simulink model "SISO_Sliding_Mode_Controlx_beta_first"  (R2021b)
settings: Solver=VariableStepAuto  StartTime=tspan(1)  StopTime=tspan(2)  RelTol=1e-8
undefined symbols (not defined in the file): BL_gain, K_switch, lambda_1_num, lambda_2_num, r_sim, Tau, y1_0, y2_0
libraries: simulink x2, simulink_extras x1
settings Model: Creator=domin  LastModifiedBy=domin
settings SolverCC: AlgebraicLoopSolver=TrustRegion
settings DebuggingCC: SFMachineParentedDataDiag=warning

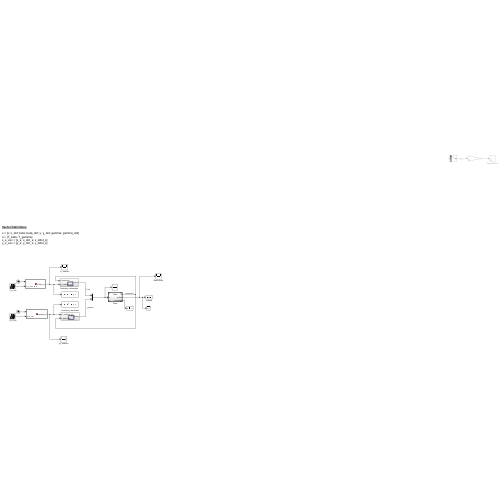
[thumbnail: Simulink's stored preview of the top-level diagram]
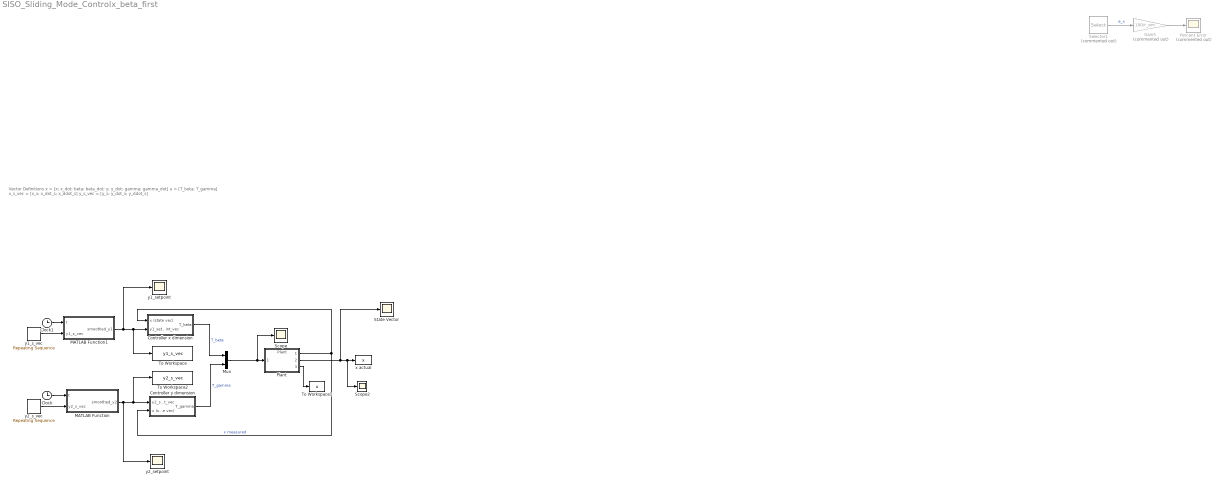
== system SISO_Sliding_Mode_Controlx_beta_first ==
  note: Vector Definitions
      |
      | x = [x; x_dot; beta; beta_dot; y; y_dot; gamma; gamma_dot]
      | u = [T_beta; T_gamma]
      | x_s_vec = [x_s; x_dot_s; x_ddot_s]
      | y_s_vec = [y_s; y_dot_s; y_ddot_s]
  Clock : Clock
  Clock1 : Clock
  Controller x dimension : Subsystem
  Controller y dimension : Subsystem
  Gain5 : Gain  Commented=on  Gain=100/r_sim
  MATLAB Function : MATLAB Function  TreatAsAtomicUnit=on
  MATLAB Function1 : MATLAB Function  TreatAsAtomicUnit=on
  Mux : Mux  Inputs=2
  Percent Error : Scope  Commented=on
  Plant : ModelReference  ModelNameDialog=Plant  SimulationMode=Normal  ModelReferenceVersion=1.107
  Scope : Scope
  Scope2 : Scope
  Selector1 : Selector  Commented=on  InputPortWidth=5  IndexOptions=Index vector (dialog)  Indices=[1]  OutputSizes=1
  State Vector : Scope
  To Workspace : ToWorkspace  VariableName=y1_s_vec  SampleTime=-1
  To Workspace1 : ToWorkspace  VariableName=u  SampleTime=-1
  To Workspace2 : ToWorkspace  VariableName=y2_s_vec  SampleTime=-1
  x actual : ToWorkspace  VariableName=x  SampleTime=-1
  y1_s_vec : simulink/Sources/Repeating Sequence  rep_seq_t=beta_BVP_sol.x'  rep_seq_y=y_s_vec_new
  y1_setpoint : Scope
  y2_s_vec : simulink/Sources/Repeating Sequence  rep_seq_t=beta_BVP_sol.x'  rep_seq_y=y_s_vec_new
  y2_setpoint : Scope
  wires:
  Gain5/1 -> Percent Error/1
  Selector1/1 -> Gain5/1  "e_x"
  Controller x dimension/1(T_beta) -> Mux/1  "T_beta"
  Controller y dimension/1(T_gamma) -> Mux/2  "T_gamma"
  Mux/1 -> Plant/1, Scope/1
  Plant/1 -> Controller x dimension/1(x (state vec)), Controller y dimension/2(x (state vec))  "x measured"
  Plant/2 -> State Vector/1, x actual/1, Scope2/1
  Plant/3 -> To Workspace1/1
  MATLAB Function/1(smoothed_y2) -> y2_setpoint/1, To Workspace2/1, Controller y dimension/1(y2_setpoint_vec)
  Clock/1 -> MATLAB Function/1(t)
  y2_s_vec/1 -> MATLAB Function/2(y2_s_vec)
  Clock1/1 -> MATLAB Function1/1(t)
  y1_s_vec/1 -> MATLAB Function1/2(y1_s_vec)
  MATLAB Function1/1(smoothed_y1) -> y1_setpoint/1, To Workspace/1, Controller x dimension/2(y1_setpoint_vec)

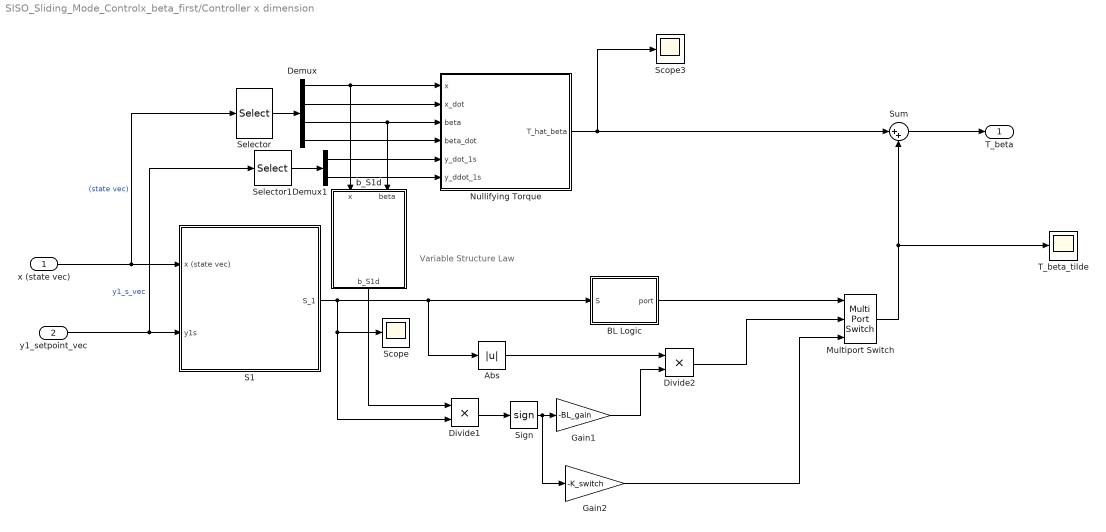
== system SISO_Sliding_Mode_Controlx_beta_first/Controller x dimension ==
  note: Variable Structure Law
  x (state vec) : Inport
  y1_setpoint_vec : Inport  Port=2
  Abs : Abs
  BL Logic : MATLAB Function  TreatAsAtomicUnit=on
  Demux : Demux
  Demux1 : Demux  Outputs=2
  Divide1 : Product  Inputs=**
  Divide2 : Product  Inputs=**
  Gain1 : Gain  Gain=-BL_gain
  Gain2 : Gain  Gain=-K_switch
  Multiport Switch : MultiPortSwitch  Inputs=2
  Nullifying Torque : MATLAB Function  TreatAsAtomicUnit=on
  S1 : Subsystem
  Scope : Scope
  Scope3 : Scope
  Selector : Selector  InputPortWidth=8  IndexOptions=Index vector (dialog)  Indices=[1:4]  OutputSizes=1
  Selector1 : Selector  InputPortWidth=3  IndexOptions=Index vector (dialog)  Indices=[2 3]  OutputSizes=1
  Sign : Signum
  Sum : Sum  Inputs=|++
  T_beta_tilde : Scope
  b_S1d : MATLAB Function  TreatAsAtomicUnit=on
  T_beta : Outport
  wires:
  Sum/1 -> T_beta/1
  x (state vec)/1 -> Selector/1, S1/1(x (state vec))  "(state vec)"
  y1_setpoint_vec/1 -> Selector1/1, S1/2(y1s)  "y1_s_vec"
  Selector/1 -> Demux/1
  Demux/2 -> Nullifying Torque/2(x_dot)
  Demux/4 -> Nullifying Torque/4(beta_dot)
  Selector1/1 -> Demux1/1
  Demux1/1 -> Nullifying Torque/5(y_dot_1s)
  Demux1/2 -> Nullifying Torque/6(y_ddot_1s)
  Nullifying Torque/1(T_hat_beta) -> Scope3/1, Sum/1
  b_S1d/1(b_S1d) -> Divide1/1
  Divide2/1 -> Multiport Switch/2
  S1/1(S_1) -> Divide1/2, Scope/1, Abs/1, BL Logic/1(S)
  Demux/3 -> Nullifying Torque/3(beta), b_S1d/2(beta)
  Demux/1 -> Nullifying Torque/1(x), b_S1d/1(x)
  Gain1/1 -> Divide2/2
  BL Logic/1(port) -> Multiport Switch/1
  Multiport Switch/1 -> Sum/2, T_beta_tilde/1
  Sign/1 -> Gain2/1, Gain1/1
  Divide1/1 -> Sign/1
  Gain2/1 -> Multiport Switch/3
  Abs/1 -> Divide2/1

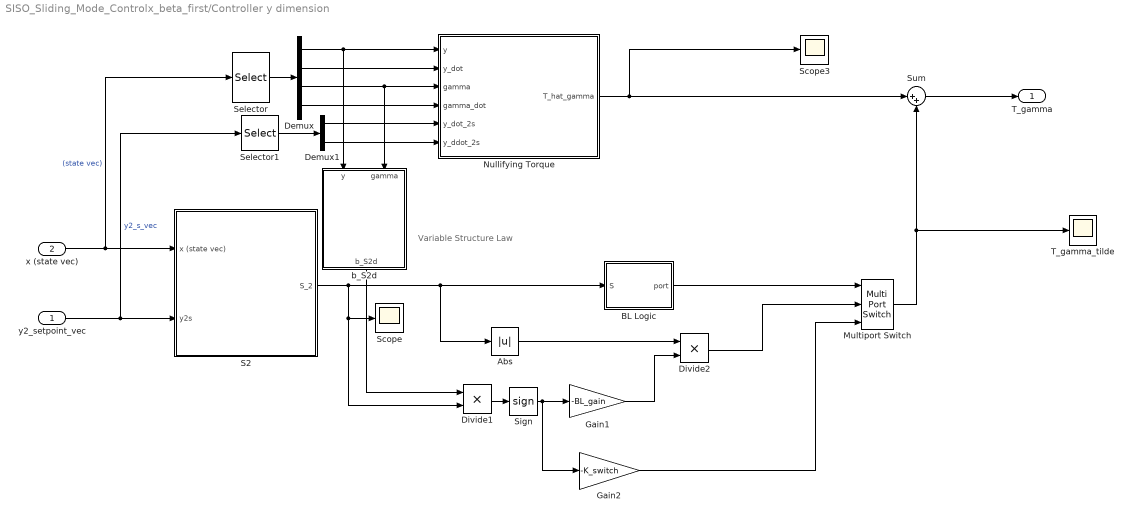
== system SISO_Sliding_Mode_Controlx_beta_first/Controller y dimension ==
  note: Variable Structure Law
  y2_setpoint_vec : Inport
  x (state vec) : Inport  Port=2
  Abs : Abs
  BL Logic : MATLAB Function  TreatAsAtomicUnit=on
  Demux : Demux
  Demux1 : Demux  Outputs=2
  Divide1 : Product  Inputs=**
  Divide2 : Product  Inputs=**
  Gain1 : Gain  Gain=-BL_gain
  Gain2 : Gain  Gain=-K_switch
  Multiport Switch : MultiPortSwitch  Inputs=2
  Nullifying Torque : MATLAB Function  TreatAsAtomicUnit=on
  S2 : Subsystem
  Scope : Scope
  Scope3 : Scope
  Selector : Selector  InputPortWidth=8  IndexOptions=Index vector (dialog)  Indices=[5:8]  OutputSizes=1
  Selector1 : Selector  InputPortWidth=3  IndexOptions=Index vector (dialog)  Indices=[2 3]  OutputSizes=1
  Sign : Signum
  Sum : Sum  Inputs=|++
  T_gamma_tilde : Scope
  b_S2d : MATLAB Function  TreatAsAtomicUnit=on
  T_gamma : Outport
  wires:
  Demux/2 -> Nullifying Torque/2(y_dot)
  Nullifying Torque/1(T_hat_gamma) -> Scope3/1, Sum/1
  Demux1/1 -> Nullifying Torque/5(y_dot_2s)
  Selector/1 -> Demux/1
  Demux/4 -> Nullifying Torque/4(gamma_dot)
  Selector1/1 -> Demux1/1
  Demux1/2 -> Nullifying Torque/6(y_ddot_2s)
  x (state vec)/1 -> Selector/1, S2/1(x (state vec))  "(state vec)"
  y2_setpoint_vec/1 -> S2/2(y2s), Selector1/1  "y2_s_vec"
  Sum/1 -> T_gamma/1
  Demux/3 -> Nullifying Torque/3(gamma), b_S2d/2(gamma)
  Demux/1 -> Nullifying Torque/1(y), b_S2d/1(y)
  Gain1/1 -> Divide2/2
  Abs/1 -> Divide2/1
  Gain2/1 -> Multiport Switch/3
  Multiport Switch/1 -> Sum/2, T_gamma_tilde/1
  BL Logic/1(port) -> Multiport Switch/1
  Sign/1 -> Gain1/1, Gain2/1
  b_S2d/1(b_S2d) -> Divide1/1
  Divide2/1 -> Multiport Switch/2
  S2/1(S_2) -> Abs/1, BL Logic/1(S), Divide1/2, Scope/1
  Divide1/1 -> Sign/1

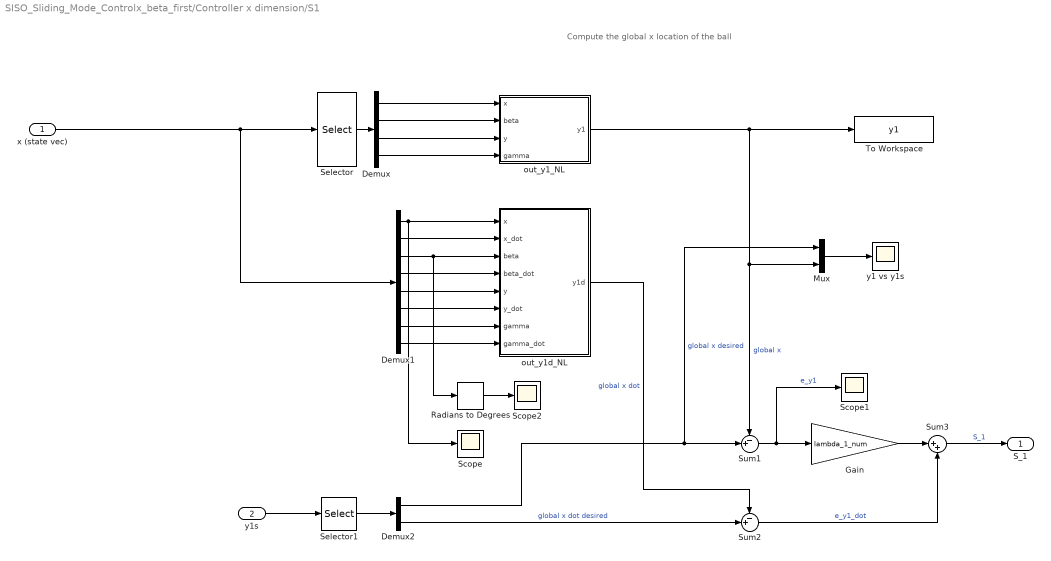
== system SISO_Sliding_Mode_Controlx_beta_first/Controller x dimension/S1 ==
  note: Compute the global x location of the ball
  x (state vec) : Inport
  y1s : Inport  Port=2
  Demux : Demux
  Demux1 : Demux  Outputs=8
  Demux2 : Demux  Outputs=2
  Gain : Gain  Gain=lambda_1_num
  Mux : Mux  Inputs=2
  Radians to Degrees : simulink_extras/Transformations/Radians to Degrees
  Scope : Scope
  Scope1 : Scope
  Scope2 : Scope
  Selector : Selector  InputPortWidth=8  IndexOptions=Index vector (dialog)  Indices=[1 3 5 7]  OutputSizes=1
  Selector1 : Selector  InputPortWidth=3  IndexOptions=Index vector (dialog)  Indices=[1 2]  OutputSizes=1
  Sum1 : Sum  Inputs=-+|
  Sum2 : Sum  Inputs=-+|
  Sum3 : Sum  Inputs=|++
  To Workspace : ToWorkspace  VariableName=y1  SampleTime=-1
  out_y1_NL : MATLAB Function  TreatAsAtomicUnit=on
  out_y1d_NL : MATLAB Function  TreatAsAtomicUnit=on
  y1 vs y1s : Scope
  S_1 : Outport
  wires:
  Demux/4 -> out_y1_NL/4(gamma)
  Sum3/1 -> S_1/1  "S_1"
  Selector/1 -> Demux/1
  Demux1/5 -> out_y1d_NL/5(y)
  Demux1/1 -> Scope/1, out_y1d_NL/1(x)
  Demux1/4 -> out_y1d_NL/4(beta_dot)
  Demux/2 -> out_y1_NL/2(beta)
  Sum1/1 -> Scope1/1, Gain/1  "e_y1"
  Sum2/1 -> Sum3/2  "e_y1_dot"
  x (state vec)/1 -> Demux1/1, Selector/1
  Gain/1 -> Sum3/1
  Demux/1 -> out_y1_NL/1(x)
  Demux/3 -> out_y1_NL/3(y)
  Demux1/2 -> out_y1d_NL/2(x_dot)
  Demux1/6 -> out_y1d_NL/6(y_dot)
  Demux1/8 -> out_y1d_NL/8(gamma_dot)
  out_y1_NL/1(y1) -> Mux/2, Sum1/1, To Workspace/1  "global x"
  Demux1/7 -> out_y1d_NL/7(gamma)
  Demux2/1 -> Mux/1, Sum1/2  "global x desired"
  Demux1/3 -> Radians to Degrees/1, out_y1d_NL/3(beta)
  Demux2/2 -> Sum2/2  "global x dot desired"
  y1s/1 -> Selector1/1
  out_y1d_NL/1(y1d) -> Sum2/1  "global x dot"
  Selector1/1 -> Demux2/1
  Mux/1 -> y1 vs y1s/1
  Radians to Degrees/1 -> Scope2/1

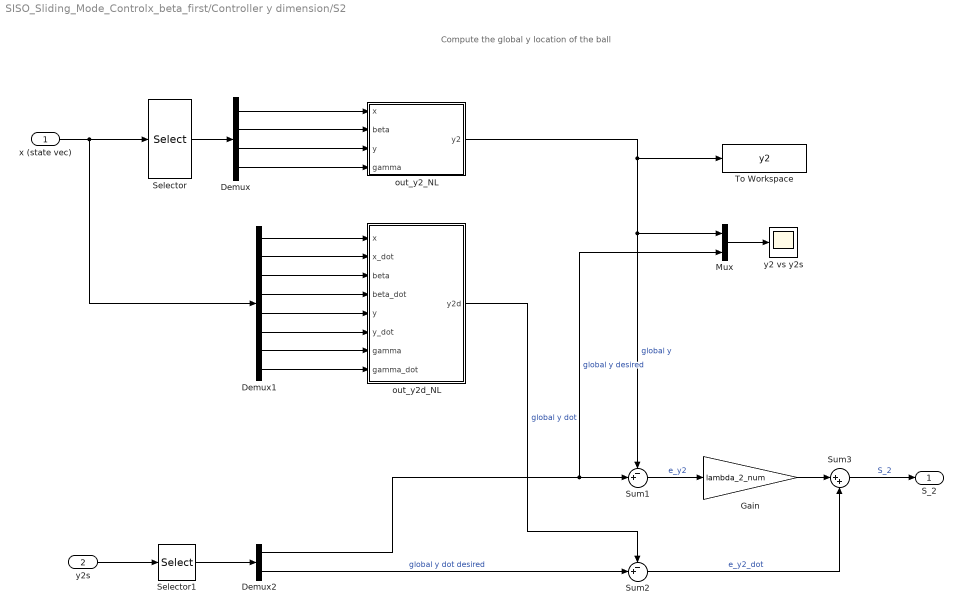
== system SISO_Sliding_Mode_Controlx_beta_first/Controller y dimension/S2 ==
  note: Compute the global y location of the ball
  x (state vec) : Inport
  y2s : Inport  Port=2
  Demux : Demux
  Demux1 : Demux  Outputs=8
  Demux2 : Demux  Outputs=2
  Gain : Gain  Gain=lambda_2_num
  Mux : Mux  Inputs=2
  Selector : Selector  InputPortWidth=8  IndexOptions=Index vector (dialog)  Indices=[1 3 5 7]  OutputSizes=1
  Selector1 : Selector  InputPortWidth=3  IndexOptions=Index vector (dialog)  Indices=[1 2]  OutputSizes=1
  Sum1 : Sum  Inputs=-+|
  Sum2 : Sum  Inputs=-+|
  Sum3 : Sum  Inputs=|++
  To Workspace : ToWorkspace  VariableName=y2  SampleTime=-1
  out_y2_NL : MATLAB Function  TreatAsAtomicUnit=on
  out_y2d_NL : MATLAB Function  TreatAsAtomicUnit=on
  y2 vs y2s : Scope
  S_2 : Outport
  wires:
  Demux/4 -> out_y2_NL/4(gamma)
  Sum3/1 -> S_2/1  "S_2"
  Selector/1 -> Demux/1
  Demux1/5 -> out_y2d_NL/5(y)
  Demux1/1 -> out_y2d_NL/1(x)
  Demux1/4 -> out_y2d_NL/4(beta_dot)
  Demux/2 -> out_y2_NL/2(beta)
  Sum1/1 -> Gain/1  "e_y2"
  Sum2/1 -> Sum3/2  "e_y2_dot"
  x (state vec)/1 -> Selector/1, Demux1/1
  Gain/1 -> Sum3/1
  Demux/1 -> out_y2_NL/1(x)
  Demux/3 -> out_y2_NL/3(y)
  Demux1/2 -> out_y2d_NL/2(x_dot)
  Demux1/6 -> out_y2d_NL/6(y_dot)
  Demux1/8 -> out_y2d_NL/8(gamma_dot)
  out_y2_NL/1(y2) -> Sum1/1, Mux/1, To Workspace/1  "global y"
  Demux1/7 -> out_y2d_NL/7(gamma)
  Demux2/1 -> Mux/2, Sum1/2  "global y desired"
  Demux1/3 -> out_y2d_NL/3(beta)
  Demux2/2 -> Sum2/2  "global y dot desired"
  y2s/1 -> Selector1/1
  out_y2d_NL/1(y2d) -> Sum2/1  "global y dot"
  Selector1/1 -> Demux2/1
  Mux/1 -> y2 vs y2s/1

== matlab function SISO_Sliding_Mode_Controlx_beta_first/Controller x dimension/S1/out_y1d_NL ==
  data: x input; y1d output; x_dot input; beta input; beta_dot input; y input; y_dot input; gamma input; gamma_dot input
function y1d = y1d(x,x_dot,beta,beta_dot,y,y_dot,gamma,gamma_dot)
%#codegen

%    This function was generated by the Symbolic Math Toolbox version 9.0.
%    16-Jan-2022 15:41:39

t2 = cos(gamma);
t3 = sin(beta);
t4 = sin(gamma);
y1d = cos(beta).*(x_dot+beta_dot.*t2.*1.406e-1+beta_dot.*t4.*y)+t2.*t3.*(gamma_dot.*y-beta_dot.*t2.*x)-t3.*t4.*(gamma_dot.*1.406e-1-y_dot+beta_dot.*t4.*x);

== matlab function SISO_Sliding_Mode_Controlx_beta_first/Controller x dimension/BL Logic ==
  data: S input; port output; S_BL_value parameter
function port = fcn(S,S_BL_value)

if abs(S) <= S_BL_value

    port = 1; %If we are in the boundary layer, use the boundary layer proportional law

else 
    port = 2; %Outside, use the signum law
end

== matlab function SISO_Sliding_Mode_Controlx_beta_first/Controller y dimension/b_S2d ==
  data: y input; b_S2d output; gamma input
function b_S2d = input_gain_S2d(y,gamma)
%#codegen

%    This function was generated by the Symbolic Math Toolbox version 9.0.
%    16-Jan-2022 15:41:42

t2 = y.^2;
t3 = t2.*(6.3e+1./4.0e+1);
t4 = t3+7.625400325243e-1;
t5 = 1.0./t4;
b_S2d = [t5.*cos(gamma).*(4.1e+1./2.0e+2)+t5.*y.*sin(gamma).*7.0];

== matlab function SISO_Sliding_Mode_Controlx_beta_first/MATLAB Function1 ==
  data: t input; y1_s_vec input; smoothed_y1 output size=2; Tau parameter; y1_0 parameter
function smoothed_y1 = fcn(t, y1_s_vec, Tau, y1_0)

smoothed_y1 = y1_s_vec*(1-exp(-t/Tau)) + y1_0*exp(-t/Tau);

== matlab function SISO_Sliding_Mode_Controlx_beta_first/MATLAB Function ==
  data: t input; y2_s_vec input; smoothed_y2 output size=2; Tau parameter; y2_0 parameter
function smoothed_y2 = fcn(t, y2_s_vec, Tau, y2_0)

smoothed_y2 = y2_s_vec*(1-exp(-t/Tau)) + y2_0*exp(-t/Tau);

== matlab function SISO_Sliding_Mode_Controlx_beta_first/Controller y dimension/S2/out_y2_NL ==
  data: x input; y2 output; beta input; y input; gamma input
function y2 = y2(x,beta,y,gamma)
%#codegen

%    This function was generated by the Symbolic Math Toolbox version 9.0.
%    16-Jan-2022 15:41:40

y2 = sin(gamma).*(-1.406e-1)+y.*cos(gamma);

== matlab function SISO_Sliding_Mode_Controlx_beta_first/Controller x dimension/S1/out_y1_NL ==
  data: x input; y1 output; beta input; y input; gamma input
function y1 = y1(x,beta,y,gamma)
%#codegen

%    This function was generated by the Symbolic Math Toolbox version 9.0.
%    16-Jan-2022 15:41:37

t2 = sin(beta);
y1 = x.*cos(beta)+t2.*cos(gamma).*1.406e-1+t2.*y.*sin(gamma);

== matlab function SISO_Sliding_Mode_Controlx_beta_first/Controller x dimension/b_S1d ==
  data: x input; b_S1d output; beta input
function b_S1d = input_gain_S1d(x,beta)
%#codegen

%    This function was generated by the Symbolic Math Toolbox version 9.0.
%    16-Jan-2022 15:41:40

t2 = x.^2;
t3 = t2.*(6.3e+1./4.0e+1);
t4 = t3+7.625400325243e-1;
t5 = 1.0./t4;
b_S1d = [t5.*cos(beta).*(-4.1e+1./2.0e+2)+t5.*x.*sin(beta).*7.0];

== matlab function SISO_Sliding_Mode_Controlx_beta_first/Controller y dimension/BL Logic ==
  data: S input; port output; S_BL_value parameter
function port = fcn(S,S_BL_value)

if abs(S) <= S_BL_value

    port = 1; %If we are in the boundary layer, use the boundary layer proportional law

else 
    port = 2; %Outside, use the signum law
end

== matlab function SISO_Sliding_Mode_Controlx_beta_first/Controller y dimension/S2/out_y2d_NL ==
  data: x input; y2d output; x_dot input; beta input; beta_dot input; y input; y_dot input; gamma input; gamma_dot input
function y2d = y2d(x,x_dot,beta,beta_dot,y,y_dot,gamma,gamma_dot)
%#codegen

%    This function was generated by the Symbolic Math Toolbox version 9.0.
%    16-Jan-2022 15:41:41

t2 = cos(gamma);
t3 = sin(gamma);
y2d = -t3.*(gamma_dot.*y-beta_dot.*t2.*x)-t2.*(gamma_dot.*1.406e-1-y_dot+beta_dot.*t3.*x);

== matlab function SISO_Sliding_Mode_Controlx_beta_first/Controller x dimension/Nullifying Torque ==
  data: x input; T_hat_beta output; x_dot input; beta input; beta_dot input; y_dot_1s input; y_ddot_1s input
function T_hat_beta = T_hat_beta(x,x_dot,beta,beta_dot,y_dot_1s,y_ddot_1s)
%#codegen

%    This function was generated by the Symbolic Math Toolbox version 9.0.
%    16-Jan-2022 15:41:39

t2 = cos(beta);
t3 = sin(beta);
t4 = beta_dot.^2;
t5 = x.^2;
t6 = t5.*(6.3e+1./4.0e+1);
t7 = t6+7.625400325243e-1;
t8 = 1.0./t7;
et1 = y_dot_1s./3.0+y_ddot_1s-beta_dot.*t2.*4.686666666666667e-2+t3.*t4.*1.406e-1-(t2.*x_dot)./3.0-t2.^2.*t8.*x.*4.5248625e-1+t3.^2.*t8.*x.*2.38889481471e+1+(beta_dot.*t3.*x)./3.0+beta_dot.*t3.*x_dot.*2.0-t2.*t3.*t8.*6.042831852210345+t2.*t4.*x+t2.*t3.*t5.*t8.*4.4145-t3.*t4.*t5.*t8.*1.7532e-1;
et2 = t2.*t4.*t8.*x.*(-5.395370803745e-1)-t2.*t4.*t8.*x.^3.*(9.0./8.0)-beta_dot.*t3.*t5.*t8.*x_dot.*(6.3e+1./2.0e+1)+beta_dot.*t2.*t8.*x.*x_dot.*9.225e-2;
T_hat_beta = (et1+et2)./(t2.*t8.*(4.1e+1./2.0e+2)-t3.*t8.*x.*7.0);

== matlab function SISO_Sliding_Mode_Controlx_beta_first/Controller y dimension/Nullifying Torque ==
  data: y input; T_hat_gamma output; y_dot input; gamma input; gamma_dot input; y_dot_2s input; y_ddot_2s input
function T_hat_gamma = T_hat_gamma(y,y_dot,gamma,gamma_dot,y_dot_2s,y_ddot_2s)
%#codegen

%    This function was generated by the Symbolic Math Toolbox version 9.0.
%    16-Jan-2022 15:41:41

t2 = cos(gamma);
t3 = sin(gamma);
t4 = gamma_dot.^2;
t5 = y.^2;
t6 = t5.*(6.3e+1./4.0e+1);
t7 = t6+7.625400325243e-1;
t8 = 1.0./t7;
et1 = y_dot_2s./3.0+y_ddot_2s+gamma_dot.*t2.*4.686666666666667e-2-t3.*t4.*1.406e-1-(t2.*y_dot)./3.0-t2.^2.*t8.*y.*4.5248625e-1+t3.^2.*t8.*y.*2.38889481471e+1+(gamma_dot.*t3.*y)./3.0+gamma_dot.*t3.*y_dot.*2.0+t2.*t3.*t8.*6.042831852210345+t2.*t4.*y-t2.*t3.*t5.*t8.*4.4145+t3.*t4.*t5.*t8.*1.7532e-1;
et2 = t2.*t4.*t8.*y.*(-5.395370803745e-1)-t2.*t4.*t8.*y.^3.*(9.0./8.0)-gamma_dot.*t3.*t5.*t8.*y_dot.*(6.3e+1./2.0e+1)-gamma_dot.*t2.*t8.*y.*y_dot.*9.225e-2;
T_hat_gamma = -(et1+et2)./(t2.*t8.*(4.1e+1./2.0e+2)+t3.*t8.*y.*7.0);
